simulink model "GFLIB_ControllerPIDpAW_BAM"  (Simulink 8.3)
settings: Solver=ode45  StartTime=0.0  StopTime=10.0  RelTol=1e-3
undefined symbols (not defined in the file): fltDerivGain, fltFiltCoef, fltIntegGain, fltPropGain
settings Model: Creator=nxf41029  LastModifiedBy=nxf41029
settings DataIOCC: SignalLoggingSaveFormat=Dataset
settings DebuggingCC: UnderspecifiedInitializationDetection=Simplified  StateNameClashWarn=none
settings GRTTargetCC: CombineOutputUpdateFcns=on  GRTInterface=off

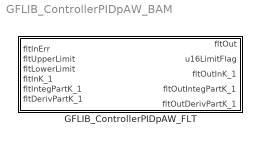
== system GFLIB_ControllerPIDpAW_BAM ==
  GFLIB_ControllerPIDpAW_FLT : Subsystem  mask(GFLIB_ControllerPIDpAW_FLT){fltPropGain=fltPropGain, fltIntegGain=fltIntegGain, fltDerivGain=fltDerivGain, fltFiltCoef=fltFiltCoef}
      mask help: Bit accurate model of parallel form PID controller. All parameters as well as input and output are single precison floating point numbers with exception of u16LimitFlag, which is 16-bit unsigned integer.
      mask init:
      | pos = get_param(gcb, 'Position');width = pos(3) - pos(1); height = pos(4) - pos(2);tX=width/2;tY=height*0.9;
      mask Display: color('black');port_label('input',1,'fltInErr');port_label('input',2,'fltUpperLimit');port_label('input',3,'fltLowerLimit');port_label('input',4,'fltInK_1');port_label('input',5,'fltIntegPartK_1');port_label('input',6,'fltDerivPartK_1');port_label('output',1,'fltOut');port_label('output',2,'u16LimitFlag');port_label('output',3,'fltOutInK_1');port_label('output',4,'fltOutIntegPartK_1');port_label('output',5,'fltOutDerivPartK_1');color('black');disp('GFLIB_ControllerPIDpAW_FLT');color('blue');text(tX,tY, 'BAM', 'horizontalAlignment', 'center');

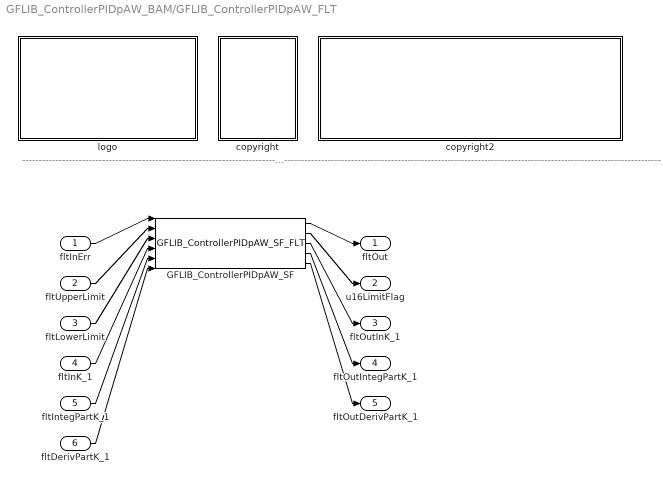
== system GFLIB_ControllerPIDpAW_BAM/GFLIB_ControllerPIDpAW_FLT ==
  note: ---------------------------------------------------------------------------------------------------------------------------------------------------------------------------------------------------
  fltInErr : Inport
  fltUpperLimit : Inport  Port=2
  fltLowerLimit : Inport  Port=3
  fltInK_1 : Inport  Port=4
  fltIntegPartK_1 : Inport  Port=5
  fltDerivPartK_1 : Inport  Port=6
  GFLIB_ControllerPIDpAW_SF : S-Function  FunctionName=GFLIB_ControllerPIDpAW_SF_FLT  Parameters=fltPropGain,fltIntegGain,fltDerivGain,fltFiltCoef  EnableBusSupport=off
  copyright : Subsystem
      mask Display: text(10,90,'FILE:');text(10,75,'DESRIPTION:');text(10,60,'COPYRIGHT:');text(10,45,'VERSION:');text(10,30,'DATE:')
  copyright2 : Subsystem
      mask Display: text(10,90,'GFLIB_ControllerPIDpAW_BAM_FLT.mdl');text(10,75,'Parallel form of a standard PID controller with implemented anti-windup.');text(10,60,'NXP');text(10,45,'0.1');text(10,30,'21-Nov-2018');
  logo : Subsystem
      mask Display: image(imread('logo.jpg'))
  fltOut : Outport
  u16LimitFlag : Outport  Port=2
  fltOutInK_1 : Outport  Port=3
  fltOutIntegPartK_1 : Outport  Port=4
  fltOutDerivPartK_1 : Outport  Port=5
  wires:
  fltInErr/1 -> GFLIB_ControllerPIDpAW_SF/1
  fltUpperLimit/1 -> GFLIB_ControllerPIDpAW_SF/2
  fltLowerLimit/1 -> GFLIB_ControllerPIDpAW_SF/3
  fltInK_1/1 -> GFLIB_ControllerPIDpAW_SF/4
  fltIntegPartK_1/1 -> GFLIB_ControllerPIDpAW_SF/5
  fltDerivPartK_1/1 -> GFLIB_ControllerPIDpAW_SF/6
  GFLIB_ControllerPIDpAW_SF/1 -> fltOut/1
  GFLIB_ControllerPIDpAW_SF/2 -> u16LimitFlag/1
  GFLIB_ControllerPIDpAW_SF/3 -> fltOutInK_1/1
  GFLIB_ControllerPIDpAW_SF/4 -> fltOutIntegPartK_1/1
  GFLIB_ControllerPIDpAW_SF/5 -> fltOutDerivPartK_1/1

== system GFLIB_ControllerPIDpAW_BAM/GFLIB_ControllerPIDpAW_FLT/copyright ==

== system GFLIB_ControllerPIDpAW_BAM/GFLIB_ControllerPIDpAW_FLT/copyright2 ==

== system GFLIB_ControllerPIDpAW_BAM/GFLIB_ControllerPIDpAW_FLT/logo ==
